simulink model "Three_Phase_Half_Wave_Rectifier_RL_Load"  (R2018a)
settings: Solver=VariableStepAuto  StartTime=0.0  StopTime=0.1  RelTol=1e-3
libraries: powerlib x16, powerlib_meascontrol x5
settings Model: Creator=ozie  LastModifiedBy=ozie

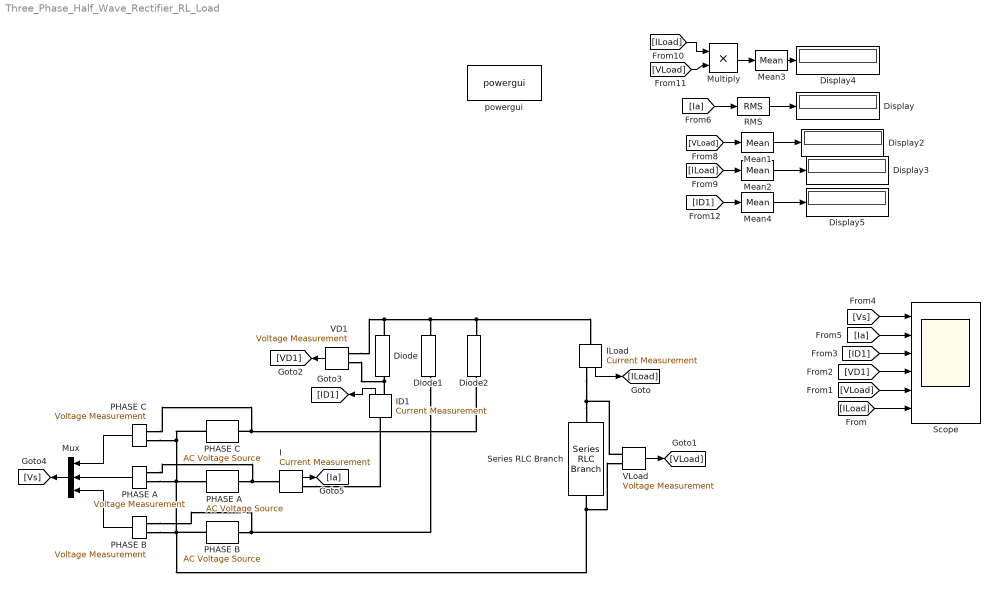
== system Three_Phase_Half_Wave_Rectifier_RL_Load ==
  Diode : powerlib/Power Electronics/Diode  Ron=0.001  Lon=0  Vf=0.8  IC=0  UseSnubber=0  Rs=500  Cs=250e-9  Measurements=on
  Diode1 : powerlib/Power Electronics/Diode  Ron=0.001  Lon=0  Vf=0.8  IC=0  UseSnubber=0  Rs=500  Cs=250e-9  Measurements=on
  Diode2 : powerlib/Power Electronics/Diode  Ron=0.001  Lon=0  Vf=0.8  IC=0  UseSnubber=0  Rs=500  Cs=250e-9  Measurements=on
  Display{,2..5} (5 alike) : Display
      Display4 settings: Format=decimal (Stored Integer)
  "I " : powerlib/Measurements/Current Measurement  PhasorSimulation=off  OutputType=Complex  PSBequivalent=0
  ID1 : powerlib/Measurements/Current Measurement  PhasorSimulation=off  OutputType=Complex  PSBequivalent=0
  ILoad : powerlib/Measurements/Current Measurement  PhasorSimulation=off  OutputType=Complex  PSBequivalent=0
  Mean{1..4} (4 alike) : powerlib_meascontrol/Measurements/Mean  Freq=50  Vinit=0  Ts=0
  Multiply : Product
  Mux : Mux  Inputs=3
      settings: DisplayOption=signals
  PHASE A : powerlib/Electrical Sources/AC Voltage Source  Amplitude=220*sqrt(2)  Phase=0  Frequency=50  SampleTime=0  Measurements=None  BusType=swing  Pref=10e3  Qref=0  Qmin=-inf  Qmax=+inf
  "PHASE A " : powerlib/Measurements/Voltage Measurement  PhasorSimulation=off  OutputType=Complex  PSBequivalent=0
  PHASE B : powerlib/Electrical Sources/AC Voltage Source  Amplitude=220*sqrt(2)  Phase=-120  Frequency=50  SampleTime=0  Measurements=None  BusType=swing  Pref=10e3  Qref=0  Qmin=-inf  Qmax=+inf
  "PHASE B " : powerlib/Measurements/Voltage Measurement  PhasorSimulation=off  OutputType=Complex  PSBequivalent=0
  PHASE C : powerlib/Measurements/Voltage Measurement  PhasorSimulation=off  OutputType=Complex  PSBequivalent=0
  "PHASE C " : powerlib/Electrical Sources/AC Voltage Source  Amplitude=220*sqrt(2)  Phase=120  Frequency=50  SampleTime=0  Measurements=None  BusType=swing  Pref=10e3  Qref=0  Qmin=-inf  Qmax=+inf
  RMS : powerlib_meascontrol/Measurements/RMS  TrueRMS=on  Freq=50  RMSInit=120  Ts=0
  Scope : Scope  NumInputPorts=6
  Series RLC Branch : powerlib/Elements/Series RLC Branch  LConnTagsString=__new0  RConnTagsString=__new0  BranchType=RL  Resistance=10  Inductance=20e-3  SetiL0=off  InitialCurrent=0  Capacitance=1e-6  Setx0=off  InitialVoltage=0  Measurements=None
  "VD1 " : powerlib/Measurements/Voltage Measurement  PhasorSimulation=off  OutputType=Complex  PSBequivalent=0
  "VLoad " : powerlib/Measurements/Voltage Measurement  PhasorSimulation=off  OutputType=Complex  PSBequivalent=0
  powergui : powerlib/powergui  Priority=1  SimulationMode=Continuous  SampleTime=50e-6  frequency=60  Iterations=50  frequencyindice=50  Pbase=100e6  ErrMax=1e-4  UnitsV=kV  UnitsW=MW  buscounter=0  FunctionMessages=off  echomessages=off  EnableUseOfTLC=off  CurrentSourceSwitches=off  DisableSnubberDevices=off  DisableRonSwitches=off  DisableVfSwitches=off  DisplayEquations=off  SolverType=Tustin/Backward Euler (TBE)  Interpol=off  ExternalGateDelay=off  methode=off  Ts=100  x0status=blocks  SPID=on  SwTol=0  HookPort=off  RestoreLinks=warning  ResistiveCurrentMeasurement=off  Frange=[0:2:500]  Ylog=off  Xlog=on  ShowGrid=off  save=off  variable=ZData  structure=0  ZoomFFT=off  StartTime=0.0  cycles=1  DisplayStyle=1  fundamental=60  FreqAxis=off  MaxFrequency=1000  frequencyindicesteady=1  RmsSteady=1  display=off
  wires:
  ILoad/1 -> [ILoad]
  "VLoad "/1 -> [VLoad]
  "VD1 "/1 -> [VD1]
  ID1/1 -> [ID1]
  PHASE C/1 -> Mux/1
  "PHASE A "/1 -> Mux/2
  "PHASE B "/1 -> Mux/3
  Mux/1 -> [Vs]
  [Vs] -> Scope/1
  "I "/1 -> [Ia]
  [Ia] -> Scope/2
  [ID1] -> Scope/3
  [VD1] -> Scope/4
  [VLoad] -> Scope/5
  [ILoad] -> Scope/6
  [Ia] -> RMS/1
  [VLoad] -> Mean1/1
  [ILoad] -> Mean2/1
  RMS/1 -> Display/1
  Mean1/1 -> Display2/1
  Mean2/1 -> Display3/1
  Multiply/1 -> Mean3/1
  [ILoad] -> Multiply/1
  [VLoad] -> Multiply/2
  Mean3/1 -> Display4/1
  [ID1] -> Mean4/1
  Mean4/1 -> Display5/1
  connections:
  ID1/RConn1 -- "VD1 "/LConn1 -- Diode/LConn1
  Series RLC Branch/LConn1 -- ILoad/RConn1 -- "VLoad "/LConn1
  PHASE A/RConn1 -- "PHASE A "/LConn1 -- "I "/LConn1
  PHASE B/RConn1 -- Diode1/LConn1 -- "PHASE B "/LConn1
  "PHASE C "/LConn1 -- PHASE C/LConn2 -- PHASE A/LConn1 -- "VLoad "/LConn2 -- Series RLC Branch/RConn1 -- "PHASE B "/LConn2 -- PHASE B/LConn1 -- "PHASE A "/LConn2
  "VD1 "/LConn2 -- Diode1/RConn1 -- Diode2/RConn1 -- ILoad/LConn1 -- Diode/RConn1
  "PHASE C "/RConn1 -- Diode2/LConn1 -- PHASE C/LConn1
  "I "/RConn1 -- ID1/LConn1
